simulink model "CML_gbyk_v4b"  (R2015a)
settings: Solver=ode4  SolverMode=MultiTasking  StartTime=0.0  StopTime=inf  FixedStep=BKIN_STEP_TIME  RelTol=1e-3
StartFcn:
  |  warndlg('Dexterit-E models cannot run under simulation. Please compile your model and run it from within Dexterit-E.');set_param(bdroot,'SimulationCommand','stop')
model workspace (MAT data in the model file):
  BKIN_STEP_TIME = 0.00025
  col_x = 1
  col_y = 2
  INIT_COLOR = 5
  DELAY_POST_TRIAL = 8
  BKIN_KINEMATIC_FRAME_SIZE = 400
  HIT_COLOR = 6
  E_NO_EVENT = 0
  START_TARGET_COL = 1
  MAX_REACH_TIME_COL = 7
  K_DELAY_FIXED = 3
  K_DELAY_RAND = 4
  K_TRIGGER_VEL = 5
  K_TRIGGER_POS = 6
  K_THRESH_VELMAX = 7
  E_NEW_TRIAL = 1
  E_STAY_START = 2
  K_REWARD_VAL = 1
  VISUAL_RADIUS = 3
  LOGICAL_RADIUS = 4
  STROKE_WIDTH = 7
  TEXT_COLOR = 8
  LABEL_HEIGHT = 10
  E_TOO_SLOW = 20
  K_SCORETEXT_ROW = 2
  LABEL = 9
  E_TARGETS_ON = 3
  DISPLAY_TRIAL_COL = 9
  E_SHOW_INSTRUCT = 13
  E_SHOW_SCORE = 14
  INSTRUCT_PAUSE_BTN = 2
  LABELONLY_X = 11
  LABELONLY_Y = 12
  K_PRE_REWARD_DELAY = 8
  CORR_TGT = 2
  INCORR_TGT = 3
  TGT_C_RWD_FRAC = 6
  BOX_HEIGHT = 13
  B1 = 10
  B2 = 11
  RWD_TARGETC1_COL = 4
  RWD_TARGETC2_COL = 5
  E_BOX_TRIGGER = 22
  E_CHOSE_ROW_B = 21
  E_HIT_TARGETB = 23
  E_MISS_TARGETB = 24
  E_HIT_TARGETC = 25
  E_MISS_TARGETC = 26
  ROTATION = 14
libraries: Video x7, slrtlib x7, KINARM_general x4, General x3, simulink x1, xpcnilib x1
CloseFcn:
  | rtwprivate ssgencode ModelCloseRequest b2lab2d
settings Model: ModifiedComment=chris -- Wed Feb 16 09:18:30 2005 -- Version 1.1384  ModifiedHistory=Feb 16/05 - Add error repeat, add offset ramp  ExtModeArmWhenConnect=off  ExtModeLogAll=off  Creator=Chris Grebeldinger  LastModifiedBy=User
settings SolverCC: EnableConcurrentExecution=on  AutoInsertRateTranBlk=on
settings DataIOCC: LimitDataPoints=off  SignalLoggingSaveFormat=ModelDataLogs  SaveOutput=off  SaveTime=off  SignalLoggingName=sigsOut
settings OptimizationCC: BlockReduction=off  BooleanDataType=off  OptimizeBlockIOStorage=off  BufferReuse=off  GlobalBufferReuse=off  ExpressionFolding=off  ExpressionDepthLimit=2147483647  LocalBlockOutputs=off  InitFltsAndDblsToZero=on
settings DebuggingCC: SaveWithParameterizedLinksMsg=none  UnderspecifiedInitializationDetection=Classic  MergeDetectMultiDrivingBlocksExec=none  SignalResolutionControl=TryResolveAllWithWarning  MultiTaskDSMMsg=warning  FcnCallInpInsideContextMsg=UseLocalSettings  StateNameClashWarn=warning  StrictBusMsg=ErrorOnBusTreatedAsVector
settings HardwareCC: ProdIntDivRoundTo=Zero  ProdEndianess=LittleEndian  ProdLongLongMode=on  ProdHWDeviceType=Generic->32-bit x86 compatible  TargetHWDeviceType=32-bit Generic
settings SFSimCC: SimCustomHeaderCode="#include \"stdlib.h\""  SFSimEcho=off  SimParseCustomCode=off
settings RTWCC: SystemTargetFile=slrt.tlc  TemplateMakefile=slrt_default_tmf  Description=Simulink Real-Time  CustomSourceCode="#include \"stdlib.h\""  RTWCompilerOptimization=on
settings CodeAppCC: MaxIdLength=63
settings SimulinkRealTimeCC: TargetFcnLib=ansi_tfl_tmw.mat  GeneratePreprocessorConditionals=Disable all  xPCisDownloadable=off  xPCisDefaultEnv=off

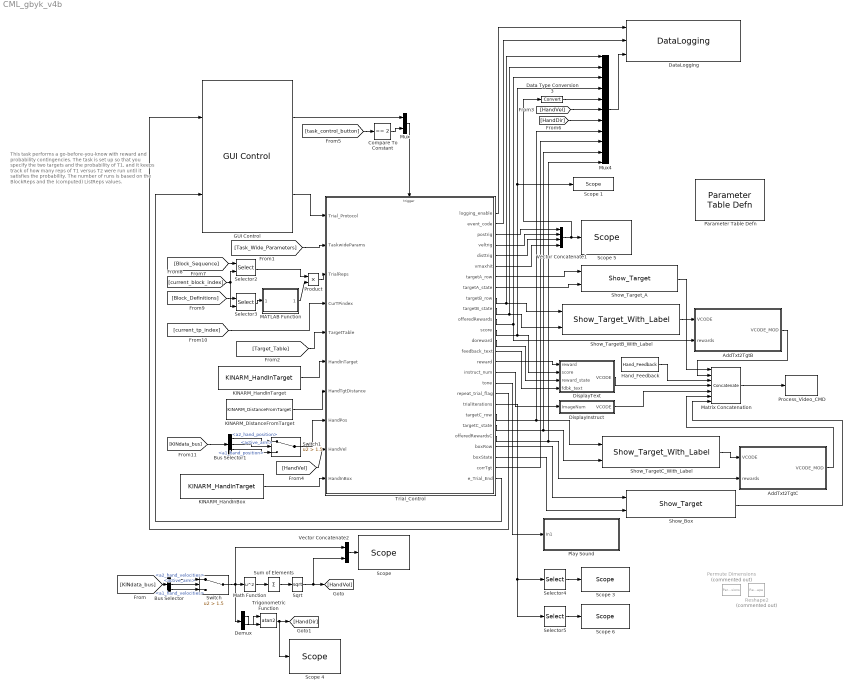
== system CML_gbyk_v4b ==
  note: This task performs a go-before-you-know with reward and probability contingencies. The task is set up so that you specify the two targets and the probability of T1, and it keeps track of how many reps of T1 versus T2 were run until it satisfies the probability. The number of runs is based on the BlockReps and the (computed) ListReps values.
  AddTxt2TgtB : MATLAB Function  TreatAsAtomicUnit=on
  AddTxt2TgtC : MATLAB Function  TreatAsAtomicUnit=on
  Bus Selector : BusSelector  OutputSignals=Robot2.a2_hand_velocities,KINDataGeneral.active_arm,Robot1.a1_hand_velocities
  Bus Selector1 : BusSelector  OutputSignals=Robot2.a2_hand_position,KINDataGeneral.active_arm,Robot1.a1_hand_position
  Compare To Constant : simulink/Logic and Bit Operations/Compare To Constant  relop===  const=2  OutDataTypeStr=boolean
  Data Type Conversion3 : DataTypeConversion
  DataLogging : General/DataLogging  log_event_codes=on  log_analog_inputs=on  show_time_remaining=off  ecat_include=on
  Demux : Demux  Outputs=2
  DisplayInstruct : Subsystem
  DisplayText : Subsystem
  GUI Control : General/GUI Control  task_version=1.0  show_repeat_trial_flag=on  use_custom_tp=off  target_type_str=Circle  Target_Type=1  XYcols=[1 2]  Vcols=3  Lcols=4  indices_padding=[0 0 0 0;0 0 0 0]  target_table_rows=32  load_table_rows=10  tp_table_rows=50
  Hand_Feedback : KINARM_general/Hand_Feedback  feedback_cntl_src=none
  KINARM_DistanceFromTarget : KINARM_general/KINARM_DistanceFromTarget  use_dominant_hand=on
  KINARM_HandInBox : KINARM_general/KINARM_HandInTarget  use_dominant_hand=on  target_type=Rectangle  num_states=1  attribcol1=[LOGICAL_RADIUS BOX_HEIGHT ROTATION]  attribcol2=[0 0 0]  attribcol3=[0 0 0]  attribcol4=[0 0 0]  attribcol5=[0 0 0]
  KINARM_HandInTarget : KINARM_general/KINARM_HandInTarget  use_dominant_hand=on  target_type=Circle  num_states=1  attribcol1=[LOGICAL_RADIUS]  attribcol2=[0]  attribcol3=[0]  attribcol4=[0]  attribcol5=[0]
  MATLAB Function : MATLAB Function  TreatAsAtomicUnit=on
  Math Function : Math  Operator=square  SaturateOnIntegerOverflow=on
  Matrix Concatenation : Concatenate  NumInputs=7  Mode=Multidimensional array
  Mux : Mux  Inputs=2
  Mux4 : Mux  Inputs=11
  Parameter Table Defn : General/Parameter Table Defn  ShowInLibBrowser=0
  Permute Dimensions : PermuteDimensions  Commented=on
  Play Sound : Subsystem
  Process_Video_CMD : Video/Process_Video_CMD  video_delay=50
  Product : Product
  Reshape2 : Reshape  Commented=on
  "Scope " : slrtlib/Displays and Logging/Scope   scopeno=1  scopetype=Target  autostart=on  viewmode=Numerical  formatstr='%15.6f'  grid=on  ylimits=[0,0]  nosamples=250  noprepostsamples=0  interleave=1  triggermode=FreeRun  triggersignal=1  trigsignalfromport=off  triggerlevel=0.0  triggerslope=Either  triggerscope=1  triggersample=0  filename=data.dat  mode=Lazy  writesize=512  autorestart=off  dynamicfilemode=off  maxwritefilesize=512*1024^2
  Scope 1 : slrtlib/Displays and Logging/Scope   scopeno=2  scopetype=Target  autostart=on  viewmode=Numerical  formatstr='%15.6f'  grid=on  ylimits=[0,0]  nosamples=250  noprepostsamples=0  interleave=1  triggermode=FreeRun  triggersignal=1  trigsignalfromport=off  triggerlevel=0.0  triggerslope=Either  triggerscope=1  triggersample=0  filename=data.dat  mode=Lazy  writesize=512  autorestart=off  dynamicfilemode=off  maxwritefilesize=512*1024^2
  Scope 3 : slrtlib/Displays and Logging/Scope   scopeno=5  scopetype=Target  autostart=on  viewmode=Numerical  formatstr='%15.6f'  grid=on  ylimits=[0,0]  nosamples=250  noprepostsamples=0  interleave=1  triggermode=FreeRun  triggersignal=1  trigsignalfromport=off  triggerlevel=0.0  triggerslope=Either  triggerscope=1  triggersample=0  filename=data.dat  mode=Lazy  writesize=512  autorestart=off  dynamicfilemode=off  maxwritefilesize=512*1024^2
  Scope 4 : slrtlib/Displays and Logging/Scope   scopeno=7  scopetype=Target  autostart=on  viewmode=Numerical  formatstr='%15.6f'  grid=on  ylimits=[0,0]  nosamples=250  noprepostsamples=0  interleave=1  triggermode=FreeRun  triggersignal=1  trigsignalfromport=off  triggerlevel=0.0  triggerslope=Either  triggerscope=1  triggersample=0  filename=data.dat  mode=Lazy  writesize=512  autorestart=off  dynamicfilemode=off  maxwritefilesize=512*1024^2
  Scope 5 : slrtlib/Displays and Logging/Scope   scopeno=8  scopetype=Target  autostart=on  viewmode=Numerical  formatstr='%15.6f'  grid=on  ylimits=[0,0]  nosamples=250  noprepostsamples=0  interleave=1  triggermode=FreeRun  triggersignal=1  trigsignalfromport=off  triggerlevel=0.0  triggerslope=Either  triggerscope=1  triggersample=0  filename=data.dat  mode=Lazy  writesize=512  autorestart=off  dynamicfilemode=off  maxwritefilesize=512*1024^2
  Scope 6 : slrtlib/Displays and Logging/Scope   scopeno=6  scopetype=Target  autostart=on  viewmode=Numerical  formatstr='%15.6f'  grid=on  ylimits=[0,0]  nosamples=250  noprepostsamples=0  interleave=1  triggermode=FreeRun  triggersignal=1  trigsignalfromport=off  triggerlevel=0.0  triggerslope=Either  triggerscope=1  triggersample=0  filename=data.dat  mode=Lazy  writesize=512  autorestart=off  dynamicfilemode=off  maxwritefilesize=512*1024^2
  Selector2 : Selector  NumberOfDimensions=2  InputPortWidth=2  IndexOptions=Index vector (port),Index vector (dialog)  Indices=2,2  OutputSizes=1,1
  Selector3 : Selector  NumberOfDimensions=2  InputPortWidth=500  IndexOptions=Index vector (port),Starting index (dialog)  Indices=2,2  OutputSizes=499,499
  Selector4 : Selector  NumberOfDimensions=2  InputPortWidth=3  IndexOptions=Select all,Index vector (dialog)  Indices=1,1  OutputSizes=1,1
  Selector5 : Selector  NumberOfDimensions=2  InputPortWidth=3  IndexOptions=Select all,Index vector (dialog)  Indices=2,2  OutputSizes=1,1
  Show_Box : Video/Show_Target  target_type=Rectangle  num_states=2  attribcol1=[0 HIT_COLOR STROKE_WIDTH VISUAL_RADIUS BOX_HEIGHT 0]  attribcol2=[HIT_COLOR HIT_COLOR STROKE_WIDTH VISUAL_RADIUS BOX_HEIGHT 0]  attribcol3=[0 0 0 0 0 0]  attribcol4=[0 0 0 0 0 0]  attribcol5=[0 0 0 0 0 0]  stateindices_padding=[0 0 0 0 0;0 0 0 0 0;0 0 0 0 0;0 0 0 0 0;0 0 0 0 0]  source=dialog  opacity=100  target_display=Both subject and operator displays  num_col=6
  Show_TargetB_With_Label : Video/Show_Target_With_Label  target_type=Circle  num_states=3  attribcol1=[0 INIT_COLOR STROKE_WIDTH VISUAL_RADIUS LABEL TEXT_COLOR LABEL_HEIGHT]  attribcol2=[INIT_COLOR INIT_COLOR STROKE_WIDTH VISUAL_RADIUS LABEL TEXT_COLOR LABEL_HEIGHT]  attribcol3=[HIT_COLOR HIT_COLOR STROKE_WIDTH VISUAL_RADIUS LABEL TEXT_COLOR LABEL_HEIGHT]  attribcol4=[0 0 0 0 0 0 0]  attribcol5=[0 0 0 0 0 0 0]  stateindices_padding=[0 0 0 0;0 0 0 0;0 0 0 0;0 0 0 0;0 0 0 0]  source=dialog  opacity=100  target_display=Both subject and operator displays
  Show_TargetC_With_Label : Video/Show_Target_With_Label  target_type=Circle  num_states=3  attribcol1=[0 INIT_COLOR STROKE_WIDTH VISUAL_RADIUS LABEL TEXT_COLOR LABEL_HEIGHT]  attribcol2=[INIT_COLOR INIT_COLOR STROKE_WIDTH VISUAL_RADIUS LABEL TEXT_COLOR LABEL_HEIGHT]  attribcol3=[HIT_COLOR HIT_COLOR STROKE_WIDTH VISUAL_RADIUS LABEL TEXT_COLOR LABEL_HEIGHT]  attribcol4=[0 0 0 0 0 0 0]  attribcol5=[0 0 0 0 0 0 0]  stateindices_padding=[0 0 0 0;0 0 0 0;0 0 0 0;0 0 0 0;0 0 0 0]  source=dialog  opacity=100  target_display=Both subject and operator displays
  Show_Target_A : Video/Show_Target  target_type=Circle  num_states=2  attribcol1=[INIT_COLOR 0 0 VISUAL_RADIUS]  attribcol2=[HIT_COLOR 0 0 VISUAL_RADIUS]  attribcol3=[0 0 0 0]  attribcol4=[0 0 0 0]  attribcol5=[0 0 0 0]  stateindices_padding=[0 0 0 0 0 0 0;0 0 0 0 0 0 0;0 0 0 0 0 0 0;0 0 0 0 0 0 0;0 0 0 0 0 0 0]  source=dialog  opacity=100  target_display=Both subject and operator displays  num_col=4
  Sqrt : Sqrt  SaturateOnIntegerOverflow=on
  Sum of Elements : Sum  Inputs=+
  Switch : Switch  Criteria=u2 > Threshold  Threshold=1.5
  Switch1 : Switch  Criteria=u2 > Threshold  Threshold=1.5
  Trial_Control : Stateflow chart  TreatAsAtomicUnit=on
  Trigonometric Function : Trigonometry  Operator=atan2  OutputSignalType=real
  Vector Concatenate1 : Concatenate  NumInputs=4  ConcatenateDimension=2
  Vector Concatenate2 : Concatenate
  wires:
  KINARM_HandInTarget/1 -> Trial_Control/6(HandInTarget)
  Show_Target_A/1 -> Matrix Concatenation/1
  GUI Control/2 -> Trial_Control/1(Trial_Protocol)
  Trial_Control/18(repeat_trial_flag) -> GUI Control/1
  Trial_Control/8(targetA_state) -> Show_Target_A/2
  Trial_Control/7(targetA_row) -> Show_Target_A/1
  Matrix Concatenation/1 -> Process_Video_CMD/1
  Hand_Feedback/1 -> Matrix Concatenation/3
  Trial_Control/9(targetB_row) -> Mux4/1, Show_TargetB_With_Label/1
  Trial_Control/10(targetB_state) -> Mux4/2, Show_TargetB_With_Label/2
  Trial_Control/1(logging_enable) -> DataLogging/1
  Trial_Control/2(event_code) -> DataLogging/2
  [KINdata_bus] -> Bus Selector/1
  KINARM_DistanceFromTarget/1 -> Trial_Control/7(HandTgtDistance)
  [Task_Wide_Parameters] -> Trial_Control/2(TaskwideParams)
  [Target_Table] -> Trial_Control/5(TargetTable)
  Trial_Control/13(doreward) -> DisplayText/3(reward_state)
  Trial_Control/26(e_Trial_End) -> GUI Control/2
  DisplayText/1(VCODE) -> Matrix Concatenation/4
  Mux4/1 -> DataLogging/3
  Trial_Control/12(score) -> Mux4/4, Scope 1/1, DisplayText/2(score)
  Trial_Control/14(feedback_text) -> DisplayText/4(fdbk_text)
  Trial_Control/3(postrig) -> Vector Concatenate1/1
  Trial_Control/4(veltrig) -> Vector Concatenate1/2
  Trial_Control/5(disttrig) -> Vector Concatenate1/3
  Trial_Control/6(vmaxhit) -> Vector Concatenate1/4
  Vector Concatenate1/1 -> Data Type Conversion3/1, Scope 5/1
  Vector Concatenate2/1 -> "Scope "/1
  Switch/1 -> Demux/1, Vector Concatenate2/1, Math Function/1
  Bus Selector/2 -> Switch/2  "<active_arm>"
  Bus Selector/3 -> Switch/3  "<a1_hand_velocities>"
  Bus Selector/1 -> Switch/1  "<a2_hand_velocities>"
  Math Function/1 -> Sum of Elements/1
  Sum of Elements/1 -> Sqrt/1
  [HandVel] -> Trial_Control/9(HandVel)
  Sqrt/1 -> Vector Concatenate2/2, [HandVel]
  Trial_Control/16(instruct_num) -> DisplayInstruct/1(ImageNum)
  DisplayInstruct/1(VCODE) -> Matrix Concatenation/5
  GUI Control/1 -> Mux/1
  [task_control_button] -> Compare To Constant/1
  Compare To Constant/1 -> Mux/2
  Mux/1 -> Trial_Control/Trigger
  Trial_Control/17(tone) -> Play Sound/1(In1)
  Demux/1 -> Trigonometric Function/2
  Demux/2 -> Trigonometric Function/1
  Trigonometric Function/1 -> Scope 4/1, [HandDir]
  [HandDir] -> Mux4/7
  Trial_Control/11(offeredRewards) -> Mux4/3, AddTxt2TgtB/2(rewards)
  [Block_Sequence] -> Selector2/1
  [current_block_index] -> Selector3/2, Selector2/2
  Selector4/1 -> Scope 3/1
  Trial_Control/19(trialIterations) -> Selector5/1, Selector4/1
  [Block_Definitions] -> Selector3/1
  Product/1 -> Trial_Control/3(TrialReps)
  Selector2/1 -> Product/1
  Selector3/1 -> MATLAB Function/1(BlockDef)
  MATLAB Function/1(ListReps) -> Product/2
  [current_tp_index] -> Trial_Control/4(CurTPindex)
  Selector5/1 -> Scope 6/1
  [HandVel] -> Mux4/6
  Bus Selector1/2 -> Switch1/2  "<active_arm>"
  Bus Selector1/3 -> Switch1/3  "<a1_hand_position>"
  Bus Selector1/1 -> Switch1/1  "<a2_hand_position>"
  [KINdata_bus] -> Bus Selector1/1
  Switch1/1 -> Trial_Control/8(HandPos)
  Show_TargetC_With_Label/1 -> AddTxt2TgtC/1(VCODE)
  Trial_Control/21(targetC_state) -> Show_TargetC_With_Label/2, Mux4/10
  Trial_Control/20(targetC_row) -> Show_TargetC_With_Label/1, Mux4/8
  Trial_Control/22(offeredRewardsC) -> AddTxt2TgtC/2(rewards), Mux4/11
  AddTxt2TgtC/1(VCODE_MOD) -> Matrix Concatenation/6
  Trial_Control/24(boxState) -> Show_Box/2
  Trial_Control/15(reward) -> DisplayText/1(reward)
  Show_TargetB_With_Label/1 -> AddTxt2TgtB/1(VCODE)
  Trial_Control/23(boxRow) -> Show_Box/1
  Show_Box/1 -> Matrix Concatenation/7
  AddTxt2TgtB/1(VCODE_MOD) -> Matrix Concatenation/2
  KINARM_HandInBox/1 -> Trial_Control/10(HandInBox)
  Data Type Conversion3/1 -> Mux4/5
  Trial_Control/25(corrTgt) -> Mux4/9

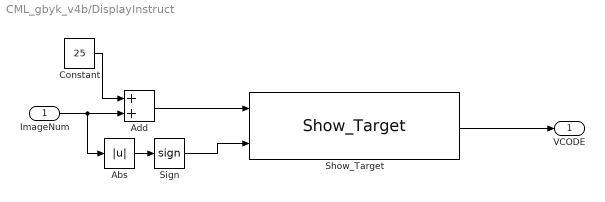
== system CML_gbyk_v4b/DisplayInstruct ==
  ImageNum : Inport
  Abs : Abs
  Add : Sum
  Constant : Constant  Value=25
  Show_Target : Video/Show_Target  target_type=Rectangle  num_states=1  attribcol1=[INIT_COLOR 0 0 VISUAL_RADIUS LABEL_HEIGHT 0]  attribcol2=[0 0 0 0 0 0]  attribcol3=[0 0 0 0 0 0]  attribcol4=[0 0 0 0 0 0]  attribcol5=[0 0 0 0 0 0]  stateindices_padding=[0 0 0 0 0;0 0 0 0 0;0 0 0 0 0;0 0 0 0 0;0 0 0 0 0]  source=dialog  opacity=100  target_display=Both subject and operator displays  num_col=6
  Sign : Signum
  VCODE : Outport
  wires:
  ImageNum/1 -> Add/2, Abs/1
  Abs/1 -> Sign/1
  Show_Target/1 -> VCODE/1
  Add/1 -> Show_Target/1
  Constant/1 -> Add/1
  Sign/1 -> Show_Target/2

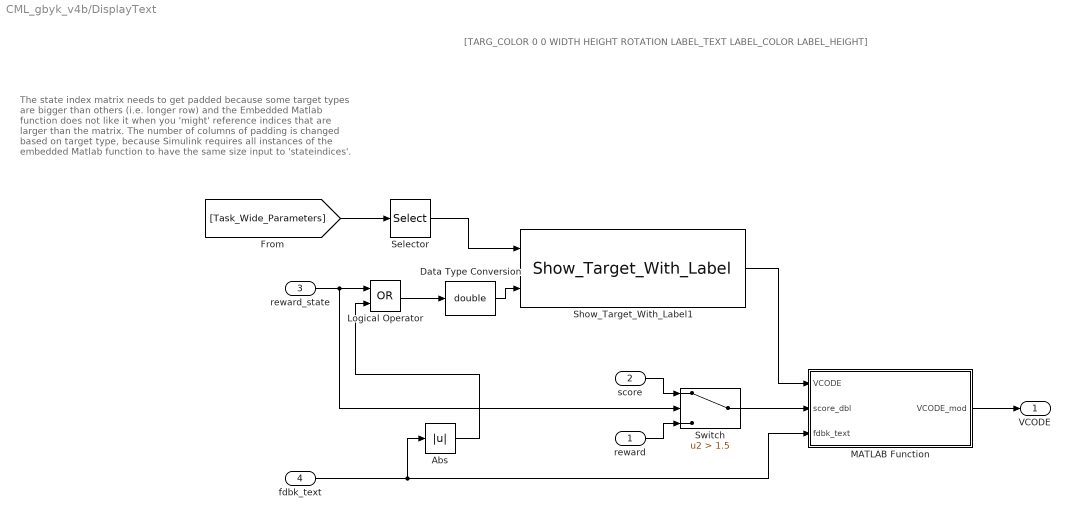
== system CML_gbyk_v4b/DisplayText ==
  note: [TARG_COLOR 0 0 WIDTH HEIGHT ROTATION LABEL_TEXT LABEL_COLOR LABEL_HEIGHT]
  note: The state index matrix needs to get padded because
      | some target types are bigger than others (i.e. longer row)
      | and the Embedded Matlab function does not like it when you
      |  'might' reference indices that are larger than the matrix.
      |
      | The number of columns of padding is changed based on target
      | type, because Simulink requires all instances of the embedded
      | Matlab function to have the same size input to 'stateindices'.
  reward : Inport
  score : Inport  Port=2
  reward_state : Inport  Port=3  OutDataTypeStr=double
  fdbk_text : Inport  Port=4  OutDataTypeStr=int32
  Abs : Abs
  Data Type Conversion : DataTypeConversion  OutDataTypeStr=double
  Logical Operator : Logic  Operator=OR  AllPortsSameDT=off  OutDataTypeStr=boolean
  MATLAB Function : MATLAB Function  TreatAsAtomicUnit=on
  Selector : Selector  InputPortWidth=50  Indices=[K_SCORETEXT_ROW]
  Show_Target_With_Label1 : Video/Show_Target_With_Label  target_type=Rectangle  num_states=1  attribcol1=[INIT_COLOR 0 0 VISUAL_RADIUS VISUAL_RADIUS 0 LABEL TEXT_COLOR LABEL_HEIGHT]  attribcol2=[0 0 0 0 0 0 0 0 0]  attribcol3=[0 0 0 0 0 0 0 0 0]  attribcol4=[0 0 0 0 0 0 0 0 0]  attribcol5=[0 0 0 0 0 0 0 0 0]  stateindices_padding=[0 0;0 0;0 0;0 0;0 0]  source=dialog  opacity=100  target_display=Both subject and operator displays
  Switch : Switch  Criteria=u2 > Threshold  Threshold=1.5
  VCODE : Outport
  wires:
  reward_state/1 -> Logical Operator/1, Switch/2
  Show_Target_With_Label1/1 -> MATLAB Function/1(VCODE)
  MATLAB Function/1(VCODE_mod) -> VCODE/1
  score/1 -> Switch/1
  reward/1 -> Switch/3
  Switch/1 -> MATLAB Function/2(score_dbl)
  [Task_Wide_Parameters] -> Selector/1
  Selector/1 -> Show_Target_With_Label1/1
  Abs/1 -> Logical Operator/2
  Logical Operator/1 -> Data Type Conversion/1
  Data Type Conversion/1 -> Show_Target_With_Label1/2
  fdbk_text/1 -> MATLAB Function/3(fdbk_text), Abs/1

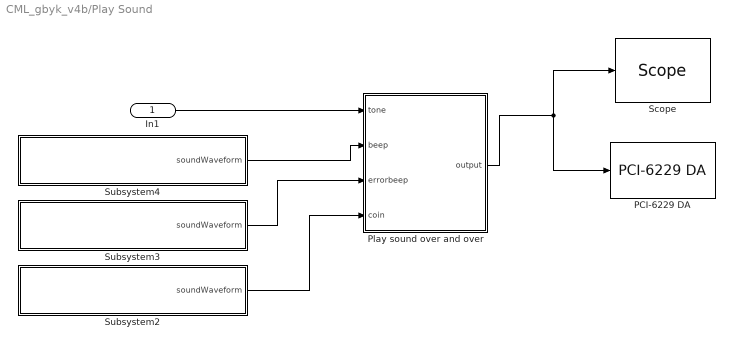
== system CML_gbyk_v4b/Play Sound ==
  In1 : Inport
  PCI-6229 DA : xpcnilib/D//A/M Series/PCI-6229 DA  channel=[1]  reset=[1]  initValue=[0]  sampletime=-1  slot=-1
  Play sound over and over : MATLAB Function  TreatAsAtomicUnit=on
  "Scope " : slrtlib/Displays and Logging/Scope   scopeno=4  scopetype=Target  autostart=on  viewmode=Graphical redraw  formatstr='%15.6f'  grid=on  ylimits=[0,0]  nosamples=4000  noprepostsamples=0  interleave=1  triggermode=FreeRun  triggersignal=1  trigsignalfromport=off  triggerlevel=0.0  triggerslope=Either  triggerscope=1  triggersample=0  filename=data.dat  mode=Lazy  writesize=512  autorestart=off  dynamicfilemode=off  maxwritefilesize=512*1024^2
  Subsystem2 : Subsystem  mask(Load Waveform Into Variable){fileName=Coin}
      mask prompts: fileName "Name of .mat Data File (must be in current directory)"
      mask help: This block will load the .MAT file specified in the dialog, and put the first variable into a GoTo called 'soundWaveform'.
      mask init:
      | filenameFromMask = get_param(gcb, 'fileName');
      | 
      | try 
      | 	dataFromFile = load(filenameFromMask);
      | 	names = fieldnames(dataFromFile);
      | 	soundDataFromFile = dataFromFile.(names{1});
      | 	display(['Sound waveform from file ''' filenameFromMask ''' loaded.']);
      | catch ME
      | 	display(ME.message)
      | end
      mask Help:
      | Enter the name a .MAT file containing a single vector or matrix. The .MAT file must be located in the current directory.
      | 
      | The first variable from the .MAT file will be put into a Goto called 'soundWaveform'.
      mask Display: disp(['Load waveform from ''' filenameFromMask ''''])
  Subsystem3 : Subsystem  mask(Load Waveform Into Variable){fileName=errorbeep}
      mask prompts: fileName "Name of .mat Data File (must be in current directory)"
      mask help: This block will load the .MAT file specified in the dialog, and put the first variable into a GoTo called 'soundWaveform'.
      mask init: same as CML_gbyk_v4b/Play Sound/Subsystem2
      mask Help:
      | Enter the name a .MAT file containing a single vector or matrix. The .MAT file must be located in the current directory.
      | 
      | The first variable from the .MAT file will be put into a Goto called 'soundWaveform'.
      mask Display: disp(['Load waveform from ''' filenameFromMask ''''])
  Subsystem4 : Subsystem  mask(Load Waveform Into Variable){fileName=beep}
      mask prompts: fileName "Name of .mat Data File (must be in current directory)"
      mask help: This block will load the .MAT file specified in the dialog, and put the first variable into a GoTo called 'soundWaveform'.
      mask init: same as CML_gbyk_v4b/Play Sound/Subsystem2
      mask Help:
      | Enter the name a .MAT file containing a single vector or matrix. The .MAT file must be located in the current directory.
      | 
      | The first variable from the .MAT file will be put into a Goto called 'soundWaveform'.
      mask Display: disp(['Load waveform from ''' filenameFromMask ''''])
  wires:
  Play sound over and over/1(output) -> PCI-6229 DA/1, "Scope "/1
  In1/1 -> Play sound over and over/1(tone)
  Subsystem2/1(soundWaveform) -> Play sound over and over/4(coin)
  Subsystem3/1(soundWaveform) -> Play sound over and over/3(errorbeep)
  Subsystem4/1(soundWaveform) -> Play sound over and over/2(beep)

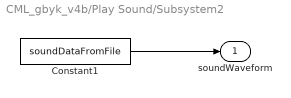
== system CML_gbyk_v4b/Play Sound/Subsystem2 ==
  Constant1 : Constant  Value=soundDataFromFile
  soundWaveform : Outport
  wires:
  Constant1/1 -> soundWaveform/1

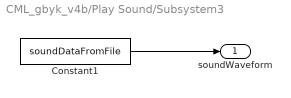
== system CML_gbyk_v4b/Play Sound/Subsystem3 ==
  Constant1 : Constant  Value=soundDataFromFile
  soundWaveform : Outport
  wires:
  Constant1/1 -> soundWaveform/1

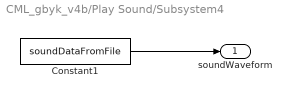
== system CML_gbyk_v4b/Play Sound/Subsystem4 ==
  Constant1 : Constant  Value=soundDataFromFile
  soundWaveform : Outport
  wires:
  Constant1/1 -> soundWaveform/1

== stateflow chart CML_gbyk_v4b/Trial_Control ==
  settings: sampleTime=0.001
  state Initialize/
    // Both the targets and data logging are initially off.
    targetA_state = 0;
    targetB_state[1] = 0;
    targetB_state[2] = 0;
    targetC_state[1] = 0;
    targetC_state[2] = 0;
    targetC_row[1] = 10;
    targetC_row[2] = 11;
    boxState = 0;
    boxRow = 8;
    logging_enable = 0;
    score = 0;
    reward = 0;
    doreward = 0;
    feedback_text = 0;
    repeat_trial_flag = 0;
    setup_trial_flag = false;
  state MainTrial
    state ShowStartTarget/
      // Turn on first target, enable data logging, and wait for a specified time or until the hand is in the target.
      targetA_row = Trial_Protocol[START_TARGET_COL];
      targetA_state = 1;
      logging_enable = 1;
      veltrig = 0;
      postrig = 0;
      disttrig = 0;
      vmaxhit = 0;
      targetB_state[1] = 0;
      targetB_state[2] = 0;
      targetC_state[1] = 0;
      targetC_state[2] = 0;
      boxState = 0;
      tone = 0;
      reward = 0;
    state SetupTgtB/
      //if turning the targets on the for the first time (each trial), set them up. We can only do this once per trial or it will throw the counters off.
      targetB_row[1] = Trial_Protocol[B1];
      targetB_row[2] = Trial_Protocol[B2];
      corrTgt = Trial_Protocol[CORR_TGT] ;
      incorrTgt = Trial_Protocol[INCORR_TGT];
      offeredRewards[1] = Trial_Protocol[RWD_TARGETC1_COL]*Trial_Protocol[TGT_C_RWD_FRAC];
      offeredRewards[2] = Trial_Protocol[RWD_TARGETC2_COL]*Trial_Protocol[TGT_C_RWD_FRAC];
      offeredRewardsC[1] = Trial_Protocol[RWD_TARGETC1_COL];
      offeredRewardsC[2] = Trial_Protocol[RWD_TARGETC2_COL];
      setup_trial_flag = true;
    state StayAtFirstTarget/
      // Log an event that target was reached and wait for a specified time.
      // The wait time may have both a fixed and a random component. The hand must stay in the target for the full wait time.
      event_code = E_STAY_START;
      targetA_state = 1;
      tickCount = TaskwideParams[K_PRE_REWARD_DELAY];
      //TODO ask aaron if we want to show the second row values too or show nothing or just what to show before the trial starts
    state ShowAllTargets/
      // Log an event that target was reached and wait for a specified time.
      // The wait time may have both a fixed and a random component. The hand must stay in the target for the full wait time.
      event_code = E_STAY_START;
      //targetA_state = 1;
      tickCount = TaskwideParams[K_DELAY_FIXED] + TaskwideParams[K_DELAY_RAND] * rand() / RAND_MAX;
      //Show targets before the go tone - allows for comparison
      targetB_state[1] = 1;
      targetB_state[2] = 1;
      targetC_state[1] = 1;
      targetC_state[2] = 1;
      boxState = 1;
    state ShowReachTargets/
      // Turn on all reach targets and log an event indicating this has occurred. Then wait until the hand is the target or until a specified time has elapsed.
      event_code = E_TARGETS_ON;
      tickCount = Trial_Protocol[MAX_REACH_TIME_COL];
      tone = 1;
      during:
      veltrig =  (HandVel > TaskwideParams[K_TRIGGER_VEL]) || veltrig;
      //postrig = abs( HandPos[1] - (TargetTable[targetA_row][col_x])) > (TargetTable[boxRow][LOGICAL_RADIUS]/2);
      //aboveasks whether the hand is past the side edges of the box which triggers rowB, this didn't work well. Below asks if hand is within some thresh distance of a rowB target
      postrig = abs(HandTgtDistance[targetB_row[1]]) < TaskwideParams[K_TRIGGER_POS]*0.01 || abs(HandTgtDistance[targetB_row[2]]) < TaskwideParams[K_TRIGGER_POS]*0.01;
      boxtrig = HandInBox[boxRow] == 1;
    state TriggerTargetC/
      event_code = E_BOX_TRIGGER;
      targetB_state[1] = 0;
      targetB_state[2] = 0;
      tone = 0;
    state TriggerTargetB/
      // if they have chosen to go for the box
      event_code = E_CHOSE_ROW_B
      tone = 0
      tgtdist = 10 + 1;// HARD CODED ( (TargetTable[targetB_row[corrTgt]][col_x] - TargetTable[targetA_row][col_x])^2.0 + (TargetTable[targetB_row[corrTgt]][col_y] - TargetTable[targetA_row][col_y])^2.0 )^0.5;
      postrig = 0;
      during:
      postrig = HandInTarget[targetB_row[corrTgt]]==1;
      tgt2trig = HandInTarget[targetB_row[incorrTgt]] ==1;
      disttrigy = (HandPos[2]) > (TargetTable[targetB_row[corrTgt]][col_y]);
      disttrig = abs(HandTgtDistance[targetA_row]) > (tgtdist)*0.01;
      disttrig = disttrig && disttrigy;
      vmaxhit = (vmaxhit || (HandVel > TaskwideParams[K_THRESH_VELMAX]));  //(sqrt(HandVel[1]^2 + HandVel[2]^2)
      minveltrig = HandVel < TaskwideParams[K_THRESH_VELMAX];
    state RevealCorrectTgtC/
      //event_code = E_CHOSE_TGT_C
      targetC_state[corrTgt] = 1;
      targetC_state[incorrTgt] = 0;
      tgtdist = 15 + 2;// if tgt xy is 25 HARD CODED because dist formula was causign problems
      during:
      //TODO fix this below
      disttrigy = (HandPos[2]) > (TargetTable[targetC_row[corrTgt]][col_y]);
      tgt2trig = HandInTarget[targetC_row[incorrTgt]] ==1;
      disttrig = abs(HandTgtDistance[targetA_row]) > (tgtdist)*0.01;
      disttrig = disttrig && disttrigy;
      postrig = HandInTarget[targetC_row[corrTgt]] ==1;
      vmaxhit = (vmaxhit || (HandVel > TaskwideParams[K_THRESH_VELMAX]));
      minveltrig = HandVel < TaskwideParams[K_TRIGGER_VEL];
    state TooSlowC/
      // Log a bad trial
      event_code = E_TOO_SLOW;
      targetC_state[1] = 0;
      targetC_state[2] = 0;
      boxState = 0;
      repeat_trial_flag = 1;
      reward = 0;
      doreward = 0;
      feedback_text = -1;
      tone = 2
      tickCount =500;
    state HitTargetC/
      // Log a successful hit
      event_code = E_HIT_TARGETC;
      targetC_state[corrTgt] = 3;
      targetC_state[incorrTgt] = 0;
      doreward = 1;
      reward = offeredRewardsC[corrTgt];
      score += reward;
      tone = 3;
      boxState = 0
      tickCount = 500;
    state MissTargetC/
      // Log a target miss
      event_code = E_MISS_TARGETC;
      targetC_state[corrTgt] = 1;
      targetC_state[incorrTgt] = 0;
      boxState =0;
      tone = 2;
      reward = 0;
      doreward = 0;
      tickCount = 500;
    state HitTargetB/
      // Log a successful hit
      event_code = E_HIT_TARGETB;
      targetB_state[corrTgt] = 3;
      targetB_state[incorrTgt] = 0;
      targetC_state[1] = 0;
      targetC_state[2] = 0;
      boxState = 0;
      doreward = 1;
      reward = offeredRewards[corrTgt];
      score += reward;
      tone = 3;
      tickCount =500;
    state MissTargetB/
      // Log a target miss
      event_code = E_MISS_TARGETB;
      targetB_state[corrTgt] = 1;
      targetB_state[incorrTgt] = 0;
      targetC_state[1] = 0;
      targetC_state[2] = 0;
      boxState = 0;
      reward = 0;
      doreward = 0;
      tone = 2;
      tickCount =500;
    state TooSlow/
      // Log a bad trial
      event_code = E_TOO_SLOW;
      targetB_state[1] = 0;
      targetB_state[2] = 0;
      targetC_state[1] = 0;
      targetC_state[2] = 0;
      boxState = 0;
      repeat_trial_flag = 1;
      reward = 0;
      doreward = 0;
      feedback_text = -1;
      tone = 2
      tickCount = 1000;
    state EndOfTrial/
      // Set the post-trial delay.
      tickCount = Trial_Protocol[DELAY_POST_TRIAL];
      boxtrig = 0;
    StayAtFirstTarget -> ShowStartTarget [order 2] : [HandInTarget[targetA_row] == 0]
    ShowStartTarget -> (junction 139)
    (junction 139) -> SetupTgtB [order 1] : [HandInTarget[targetA_row] == 1 && !setup_trial_flag]
    (junction 139) -> StayAtFirstTarget [order 2] : [HandInTarget[targetA_row] == 1 && setup_trial_flag]
    SetupTgtB -> StayAtFirstTarget
    StayAtFirstTarget -> ShowAllTargets [order 1] : after(tickCount, e_clk)
    ShowAllTargets -> ShowReachTargets : after(tickCount,e_clk)
    ShowReachTargets -> TooSlow [order 1] : after(tickCount, e_clk)/
        | feedback_text = -2;
        | //if the trial times out it is an error
    ShowReachTargets -> TriggerTargetC [order 3] : [after(1,e_clk) && veltrig && boxtrig]
    ShowReachTargets -> TriggerTargetB [order 2] : [after(1,e_clk) && veltrig && postrig && !boxtrig]
    TriggerTargetC -> RevealCorrectTgtC : after(1,e_clk)
    TriggerTargetB -> TooSlow [order 1] : [(after(1,e_clk) && (disttrig || postrig) && vmaxhit == 0) || minveltrig || after(tickCount, e_clk)]/
        | feedback_text = -1;
        | //check if missed the target but moved fast enough
    RevealCorrectTgtC -> TooSlowC [order 1] : [(after(1,e_clk) && (disttrig || postrig) && vmaxhit == 0) || minveltrig || after(tickCount, e_clk)]
        | //check if missed the target but moved fast enough
    TriggerTargetB -> HitTargetB [order 3] : [after(1,e_clk) && postrig && vmaxhit]
        | //check if hit the target and moved fast enough
    TriggerTargetB -> MissTargetB [order 2] : [after(1,e_clk) && (tgt2trig || (disttrig && !postrig)) && vmaxhit]/
        | //check if missed the target but moved fast enough
    RevealCorrectTgtC -> MissTargetC [order 3] : [after(1,e_clk) && (tgt2trig || (disttrig && !postrig)) && vmaxhit]/
        | //check if missed the target but moved fast enough
    RevealCorrectTgtC -> HitTargetC [order 2] : [after(1,e_clk) && postrig && vmaxhit]
        | //check if hit the target and moved fast enough
    TooSlowC -> EndOfTrial
    MissTargetC -> EndOfTrial
    HitTargetC -> EndOfTrial
    HitTargetB -> EndOfTrial : after(tickCount, e_clk)
    MissTargetB -> EndOfTrial : after(tickCount, e_clk)
    TooSlow -> EndOfTrial : after(tickCount, e_clk)
  state EndInstructPause/
    instruct_num = 0;
    tickCount = Trial_Protocol[DELAY_POST_TRIAL];
    logging_enable = 1;
    score = 0;
  state Ending/
    //end the special "show score" state
    //score = 0;
    e_Trial_End;
  state ReturnToStart1/
    targetA_state=1;
    targetB_state[1] = 0;
    targetB_state[2] = 0;
    targetC_state[1] = 0;
    targetC_state[2] = 0;
    boxState = 0;
    feedback_text = 0;
    doreward = 0;
    repeat_trial_flag = 0;
    logging_enable = 1;
    setup_trial_flag = false;
  state InstructWaitState/
    //"pause" here until the button has been clicked
  state ShowScoreState/
    event_code = E_SHOW_SCORE;
    targetA_state = 0;
    targetB_state[1] = 0;
    targetB_state[2] = 0;
    targetC_state[1] = 0;
    targetC_state[2] = 0;
    boxState = 0;
    doreward = 2;
    tickCount = 10000;
    logging_enable = 0;
  state ShowInstructState/
    event_code = E_SHOW_INSTRUCT;
    targetA_state = 0;
    targetB_state[1] = 0;
    targetB_state[2] = 0;
    targetC_state[1] = 0;
    targetC_state[2] = 0;
    boxState = 0;
    doreward = 0;
    instruct_num = Trial_Protocol[DISPLAY_TRIAL_COL];
    tickCount = Trial_Protocol[MAX_REACH_TIME_COL];
    logging_enable = 0;
  state Inter_Trial_State/
    // Turn off both targets, turn off data logging, reset the
    // event code, and send the e_Trial_End Stateflow event.
    event_code = 0;
    targetA_state = 1;
    targetB_state[1] = 0;
    targetB_state[2] = 0;
    targetC_state[1] = 0;
    targetC_state[2] = 0;
    boxState = 0;
    offeredRewards[1] = 0;
    offeredRewards[2] = 0;
    feedback_text = 0;
    doreward = 0;
    setup_trial_flag = false;
    veltrig = 0;
    vmaxhit = 0;
    postrig = 0;
    boxtrig = 0;
    tgt2trig = 0;
    disttrig = 0;
    minveltrig = 0;
    disttrigy = 0;
    e_Trial_End;
  (default) -> Initialize
  Initialize -> ShowStartTarget [order 1] : [Trial_Protocol[DISPLAY_TRIAL_COL] == 0]
  ReturnToStart1 -> ShowStartTarget : after(1, e_clk)/
  Initialize -> ShowInstructState [order 2] : [Trial_Protocol[DISPLAY_TRIAL_COL] > 0]
      | //in case we start with an instruction trial
  Ending -> (junction 91) : after(1,e_clk)
  (junction 91) -> EndInstructPause [order 1] : [Trial_Protocol[DISPLAY_TRIAL_COL] == 0]/
      | //continue if a regular trial comes after!
  (junction 91) -> ShowInstructState [order 2] : //so we can show the score and then show instructions
      | [Trial_Protocol[DISPLAY_TRIAL_COL] > 0]
  EndInstructPause -> ReturnToStart1 : after(tickCount,e_clk)
  InstructWaitState -> Ending : e_cntl_btn/
      | event_code = 22;
  ShowScoreState -> Ending : after(tickCount,e_clk)
  ShowInstructState -> InstructWaitState : after(tickCount,e_clk)
  (junction 86) -> ReturnToStart1 [order 3] : [Trial_Protocol[DISPLAY_TRIAL_COL] == 0]
  (junction 86) -> ShowScoreState [order 1] : [Trial_Protocol[DISPLAY_TRIAL_COL] == -1]
  (junction 86) -> ShowInstructState [order 2] : [Trial_Protocol[DISPLAY_TRIAL_COL] > 0]
  Inter_Trial_State -> (junction 86) : after(1,e_clk)
  MainTrial -> Inter_Trial_State : e_ExitTrialNow/
      | tickCount = 1;
  EndOfTrial -> Inter_Trial_State : after(tickCount,e_clk)
  data: logging_enable output double size=1; Trial_Protocol input double size=50; TaskwideParams input double; TrialReps input double; CurTPindex input; TargetTable input double; HandInTarget input double; event_code output uint16 [0..] =0; postrig output boolean; veltrig output boolean; disttrig output boolean; vmaxhit output boolean; targetA_row output [1..32]; targetA_state output double; targetB_row output double size=[2]; targetB_state output double size=[2]; offeredRewards output double size=2; score output double; tickCount local double; RAND_MAX constant double =32767; HandTgtDistance input double; HandPos input double; HandVel input double; doreward output double; feedback_text output int32; reward output double; instruct_num output double; tone output double; repeat_trial_flag output double; tgtdist local double; trialIterations output double size=[60, 2] =0; targetC_row output double size=[2]; targetC_state output double size=[2]; offeredRewardsC output double size=[2]; boxRow output double size=1; rwdTgts local double size=2; pTgts local double size=2; setup_trial_flag local boolean; disttrigy local boolean; tgt2trig local double; boxState output double size=1; corrTgt output double; incorrTgt local double; boxtrig local double; HandInBox input double; minveltrig local double
  data targetA_row settings: description=index of the row currently being used in the TargetTable
  events: e_clk input RISING_EDGE_EVENT; e_ExitTrialNow input EITHER_EDGE_EVENT; e_Trial_End output EITHER_EDGE_EVENT; e_cntl_btn input EITHER_EDGE_EVENT

== matlab function CML_gbyk_v4b/AddTxt2TgtB ==
  data: VCODE input; VCODE_MOD output; rewards input
function VCODE_MOD  = rwd_tgt(VCODE,rewards)
%#codegen

VCODE_MOD = VCODE;

%rewards = rwd_multipliers*rwd_val;

for a = 1:length(rewards)

    if any(rewards)>0
        jj = 1;
        label = rewards(a);
        
        if (label < 10)
            VCODE_MOD(a, jj + 14) = int32(label+int32('0'));
            
        elseif (label < 100) %score < $1
            n1 = int32(floor(double(label)/10));  %we need to cast score to a double otherwise the arithmetic is wrong!
            n2 = label - n1*10;
        
            VCODE_MOD(a, jj + 14) = int32(n1+int32('0'));
            jj = jj+1;
            VCODE_MOD(a, jj + 14) = int32(n2+int32('0'));
        else %label < 1000
            n1 = int32(floor(double(label)/100));  %we need to cast score to a double otherwise the arithmetic is wrong!
            n2 = label - n1*100;
            n2 = int32(floor(double(n2)/100));  %we need to cast score to a double otherwise the arithmetic is wrong!
            n3 = label - n1*100 - n2*10;
        
            VCODE_MOD(a, jj + 14) = int32(n1+int32('0'));
            jj = jj+1;
            VCODE_MOD(a, jj + 14) = int32(n2+int32('0'));
            jj = jj+1;
            VCODE_MOD(a, jj + 14) = int32(n3+int32('0'));
        end
        VCODE_MOD(a,jj + 1 + 14) = 0; %terminate string
    else
        VCODE_MOD(a,15) = 0; %terminate string
    end
end

== matlab function CML_gbyk_v4b/Play Sound/Play sound over and over ==
  data: tone input; output output; beep input; errorbeep input; coin input
function output = fcn(tone,beep,errorbeep,coin)
%#codegen

persistent t last_tone_state
if isempty(t), t = 0; end
if isempty(last_tone_state), last_tone_state = 0; end

trigger = last_tone_state ~= tone;
if trigger > 0
    last_tone_state = tone;
end

output = 0;		% default
if t == 0 && trigger > 0
	% start the playing of the sound.
	t = t + 1;
end

if tone == 1
    data = beep;
elseif tone == 2
    data = errorbeep;
elseif tone == 3
    data = coin;
else 
    t = 0;
    data = 0;
end

if t > 0
	output = data(t);
	if t == length(data)
		t = 0;
	else
		t = t + 1;
	end
end

== matlab function CML_gbyk_v4b/MATLAB Function ==
  data: BlockDef input; ListReps output
function ListReps = calcListReps(BlockDef)
%#codegen

BlockDef = nonzeros(BlockDef);
%BlockDef = BlockDef(2:end);

trials = unique(BlockDef);
reps1 = sum(BlockDef == trials(1));
reps2 = sum(BlockDef == trials(2));
reps3 = sum(BlockDef == trials(3));
ListReps = round(mean([reps1,reps2,reps3]));

== matlab function CML_gbyk_v4b/DisplayText/MATLAB Function ==
  data: VCODE input; score_dbl input; VCODE_mod output; fdbk_text input
function VCODE_mod = fcn(VCODE,score_dbl,fdbk_text)


VCODE_mod = VCODE;

score = round(score_dbl);  %for display purposes, round fractional rewards

if (fdbk_text == 0)  %if this is zero, show the score
       
    
    %score is in cents. potentially need to convert to dollars
    
    if (score < 10)
        text1 = 'You earned ';
        text2 = ' cents!';
        
        textout = [text1 int2char(int32(score)) text2];
        
    elseif (score < 100) %score < $1
        text1 = 'You earned ';
        text2 = ' cents!';
        
        n1 = int32(floor(double(score)/10));  %we need to cast score to a double otherwise the arithmetic is wrong!
        n2 = score - n1*10;
        
        textout = [text1 int2char(int32(n1)) int2char(int32(n2)) text2];
        
    else %score > $1, convert to dollars to keep the score readable
        text1 = 'You earned $';
        text2 = '.';
        text3 = '!';
        
        dollars = int32(floor(double(score)/100));
        if (dollars >= 10) %double digit dollar value
            n1d = int32(floor(double(dollars)/10));
            n2d = dollars - n1d*10;
            textdollars = [int2char(int32(n1d)) int2char(int32(n2d))];
        else %single digit
            textdollars = int2char(int32(dollars));
        end
        
        cents = score-dollars*100;
        if (cents < 10)
            textcents = ['0' int2char(int32(cents))];
        else
            n1 = int32(floor(double(cents)/10));
            n2 = round(cents - n1*10);
            textcents = [int2char(int32(n1)) int2char(int32(n2))];
        end
        
        textout = [text1 textdollars text2 textcents text3];
        
    end
    
elseif (fdbk_text == 1) 
    %print "too fast"
    textout = 'Too Fast!';
    
    
elseif (fdbk_text == 2) 
    %print "too fast"
    textout = 'Too Early!';

elseif (fdbk_text == -1) 
    %print "too slow"
    
    textout = 'Too Slow!';

elseif (fdbk_text == -2) 
    %print "too fast"
    textout = 'Too Late!';


else
    textout = '';
    
end
    

%the first character is VCODE(15)
%need to translate text into ascii:
textnum = double(textout); %this quickly casts each char into a number

%make sure we won't overflow the VCODE: no more than 50 chars! we will
%clip off anything that overflows.
VCODE_mod(1,15:min([15+length(textout),64])) = textnum(1:min([length(textnum),50])); %write out as many the characters as possible into the VCODE
VCODE_mod(1,min([15+length(textout)+1,64])) = 0;  %terminate the string!



function s = int2char(n)

n = mod(n,10); %make sure we only have 1 digit or we will get a weird character!

s = char(n+int32('0')); %// add the character

== matlab function CML_gbyk_v4b/AddTxt2TgtC ==
  data: VCODE input; VCODE_MOD output; rewards input
function VCODE_MOD  = rwd_tgt(VCODE,rewards)
%#codegen

VCODE_MOD = VCODE;

%rewards = rwd_multipliers*rwd_val;

for a = 1:length(rewards)

    if any(rewards)>0
        jj = 1;
        label = rewards(a);
        
        if (label < 10)
            VCODE_MOD(a, jj + 14) = int32(label+int32('0'));
            
        elseif (label < 100) %score < $1
            n1 = int32(floor(double(label)/10));  %we need to cast score to a double otherwise the arithmetic is wrong!
            n2 = label - n1*10;
        
            VCODE_MOD(a, jj + 14) = int32(n1+int32('0'));
            jj = jj+1;
            VCODE_MOD(a, jj + 14) = int32(n2+int32('0'));
        else %label < 100
            n1 = int32(floor(double(label)/100));  %we need to cast score to a double otherwise the arithmetic is wrong!
            n2 = label - n1*100;
            n2 = int32(floor(double(n2)/100));  %we need to cast score to a double otherwise the arithmetic is wrong!
            n3 = label - n1*100 - n2*10;
        
            VCODE_MOD(a, jj + 14) = int32(n1+int32('0'));
            jj = jj+1;
            VCODE_MOD(a, jj + 14) = int32(n2+int32('0'));
            jj = jj+1;
            VCODE_MOD(a, jj + 14) = int32(n3+int32('0'));
        end
        VCODE_MOD(a,jj + 1 + 14) = 0; %terminate string
    else
        VCODE_MOD(a,15) = 0; %terminate string
    end
end
